simulink subsystem "HallSensor"  (R2025a)
settings: Solver=VariableStepAuto  StartTime=0.0  StopTime=10.0  RelTol=1e-3
model mask{kw=0, kphi=0}
settings Model: Creator=Глеб  LastModifiedBy=Глеб

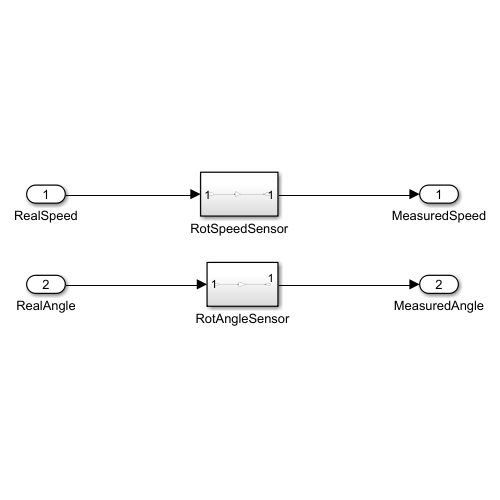
[thumbnail: Simulink's stored preview of the top-level diagram]
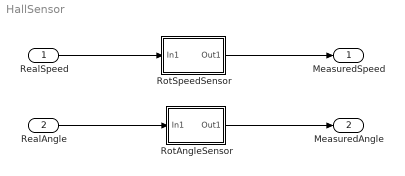
== system HallSensor ==
  RealSpeed : Inport
  RealAngle : Inport  Port=2
  RotAngleSensor : Subsystem
  RotSpeedSensor : Subsystem
  MeasuredSpeed : Outport
  MeasuredAngle : Outport  Port=2
  wires:
  RealAngle/1 -> RotAngleSensor/1(In1)
  RotSpeedSensor/1(Out1) -> MeasuredSpeed/1
  RotAngleSensor/1(Out1) -> MeasuredAngle/1
  RealSpeed/1 -> RotSpeedSensor/1(In1)

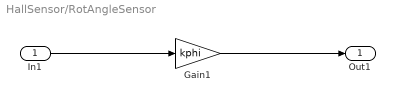
== system HallSensor/RotAngleSensor ==
  In1 : Inport
  Gain1 : Gain  Gain=kphi
  Out1 : Outport
  wires:
  In1/1 -> Gain1/1
  Gain1/1 -> Out1/1

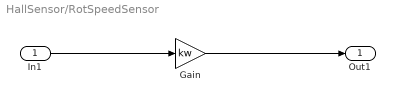
== system HallSensor/RotSpeedSensor ==
  In1 : Inport
  Gain : Gain  Gain=kw
  Out1 : Outport
  wires:
  In1/1 -> Gain/1
  Gain/1 -> Out1/1
